simulink model "Test_neural_2017a"  (R2017a)
settings: Solver=FixedStepAuto  StartTime=0.0  StopTime=tf  FixedStep=0.001  RelTol=1e-3
undefined symbols (not defined in the file or in its folder): Continuous, Time
libraries: neural x37, ctrlSharedLib x2
(part 2 of 2)

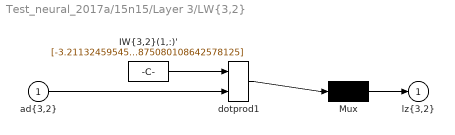
== system Test_neural_2017a/15n15/Layer 3/LW{3,2} ==
  "ad{3,2}" : Inport  PortDimensions=15
      mask Display: e = 0.06;c1 = [120 230 180]/255;c2 = ([120 230 180]+0)/(256+128);c3 = ([120 230 180]+128)/(256+128);patch([0 1 1 0],[0 0 1 1],c1);patch([0 1 1 1-e 1-e 0+e],[0 0 1 1-e 0+e 0+e],c2);patch([0 0 1 1-e 0+e 0+e],[0 1 1 1-e 1-e 0+e],c3);plot([0 1 1 0 0],[0 0 1 1 0]);
  "IW{3,2}(1,:)'" : Constant  Value=[-3.21132459545898729658119918894954025745391845703125;10.2228101765280836588090096483938395977020263671875;-0.93380636270399663967367587247281335294246673583984375;1.4919199213879739129851031975704245269298553466796875;1.306433261350524954735874416655860841274261474609375;4.17931555842425783708904418745078146457672119140625;-3.251465482956536590108953532762825489044189453125;11.323555323158263519189858925528824329376220703125;-1.2967491227195815373107734558288939297199249267578125;-10.8432048609134294991918068262748420238494873046875;4.259778382156749643172588548623025417327880859375;3.05232059391192489528066289494745433330535888671875;7.276161239460694929448436596430838108062744140625;0.64954130325699421799612309769145213067531585693359375;-1.5996298779181110649716401894693262875080108642578125]
      mask Display: e = 0.06;c1 = [120 150 230]/255;c2 = ([120 150 230]+0)/383;c3 = ([120 150 230]+128)/383;patch([0 1 1 0],[0 0 1 1],c1);patch([0 1 1 1-e 1-e 0+e],[0 0 1 1-e 0+e 0+e],c2);patch([0 0 1 1-e 0+e 0+e],[0 1 1 1-e 1-e 0+e],c3);plot([0 1 1 0 0],[0 0 1 1 0]);disp('weights');
  Mux : Mux  Inputs=1
      mask Display: e = 0.06;c1 = [120 150 230]/255;c2 = ([120 150 230]+0)/383;c3 = ([120 150 230]+128)/383;patch([0 1 1 0],[0 0 1 1],c1);patch([0 1 1 1-e 1-e 0+e],[0 0 1 1-e 0+e 0+e],c2);patch([0 0 1 1-e 0+e 0+e],[0 1 1 1-e 1-e 0+e],c3);plot([0 1 1 0 0],[0 0 1 1 0]);disp('Mux');
  dotprod1 : neural/Weight Functions/dotprod
  "lz{3,2}" : Outport
      mask Display: e = 0.06;c1 = [120 230 180]/255;c2 = ([120 230 180]+0)/(256+128);c3 = ([120 230 180]+128)/(256+128);patch([0 1 1 0],[0 0 1 1],c1);patch([0 1 1 1-e 1-e 0+e],[0 0 1 1-e 0+e 0+e],c2);patch([0 0 1 1-e 0+e 0+e],[0 1 1 1-e 1-e 0+e],c3);plot([0 1 1 0 0],[0 0 1 1 0]);
  wires:
  "IW{3,2}(1,:)'"/1 -> dotprod1/1
  "ad{3,2}"/1 -> dotprod1/2
  dotprod1/1 -> Mux/1
  Mux/1 -> "lz{3,2}"/1

== matlab function Test_neural_2017a/ZeroandHold/MATLAB Function ==
  data: a input; z1 input; y1 input; clock input; u input; n11 input; y output; n1 output
function [y,n1] = fcn(a,z1,y1,clock,u,n11)
dt = 0.001;
n = clock/dt;
if z1<0
    y =0;
    n1=n;
else
    if z1 == 0
        n1 = n;
    else 
        n1 = n11;
    end
    if n<n1+300
        deln = n-n1;
        if rem(deln,a)==0
            y = u;
        else
            y = y1;
        end
    else
        y=0;
    end
end
